simulink model "Aircraft_Simulator_final_"  (R2019b)
settings: Solver=ode4  StartTime=0.0  StopTime=tfinal  FixedStep=dt  RelTol=1e-3
values from neighbouring files (symbols this model uses):
  A_2D = [Yv, -(1-Yr/u0) ... (first row only)    [Approximations.m]
  A_DR = [Yv, 0, -1 ... (first row only)    [Approximations.m]
  A_FL = [Xu, Xw, -w0, -g*cos(theta0) ... (first row only)    [Approximations.m]
  A_lat = [Yb/Vto, (Yp+w0)/Vto, (Yr-u0)/Vto, (g*cos(theta0))/Vto, 0 ... (first row only)    [Approximations.m]
  A_LP = [Xu+w0*Zu/(Zq+u0),          -g*cos(theta0)-w0*g*sin(theta0)/(Zq+u0) ... (first row only)    [Approximations.m]
  A_RO = [Lp_dash]    [Approximations.m]
  A_SP = [Zw/(1-Zwdot), (Zq+u0)/(1-Zwdot) ... (first row only)    [Approximations.m]
  A_Sp = [Lp_dash, Lr_dash, 0 ... (first row only)    [Approximations.m]
  B_2D = [Yda_star, Ydr_star ... (first row only)    [Approximations.m]
  B_DR = [Yda_star, Ydr_star ... (first row only)    [Approximations.m]
  B_FL = [Xde, Xdth ... (first row only)    [Approximations.m]
  B_lat = [Yda_star, Ydr_star ... (first row only)    [Approximations.m]
  B_LP = [Xde+w0*Zde/(Zq+u0), Xdth+w0*Zdth/(Zq+u0) ... (first row only)    [Approximations.m]
  B_RO = [Lda_dash]    [Approximations.m]
  B_SP = [Zde/(1-Zwdot), Zdth/(1-Zwdot) ... (first row only)    [Approximations.m]
  B_Sp = [Lda_dash  Ldr_dash ... (first row only)    [Approximations.m]
  C_2D = eye(2)    [Approximations.m]
  C_DR = eye(3)    [Approximations.m]
  C_FL = eye(4)    [Approximations.m]
  C_lat = eye(5)    [Approximations.m]
  C_LP = eye(2)    [Approximations.m]
  C_RO = eye(1)    [Approximations.m]
  C_SP = eye(2)    [Approximations.m]
  C_Sp = eye(3)    [Approximations.m]
  D_2D = zeros(2)    [Approximations.m]
  D_DR = zeros(3,2)    [Approximations.m]
  D_FL = zeros(4,2)    [Approximations.m]
  D_lat = zeros(5,2)    [Approximations.m]
  D_LP = zeros(2)    [Approximations.m]
  D_RO = zeros(1)    [Approximations.m]
  D_SP = zeros(2,2)    [Approximations.m]
  D_Sp = zeros(3,2)    [Approximations.m]
  da = da(k)*pi/180    [Task4MainCode.m]
  de = 0    [Task4MainCode.m]
  dr = dr(k)*pi/180    [Task4MainCode.m]    (also in afModel.m = cuStates(6)-states0(6))
  dth = 0    [Task4MainCode.m]
undefined symbols (not defined in the file or in its folder): aircraft_data, s0
settings Model: Creator=yossef  LastModifiedBy=Yousef
settings DataIOCC: ReturnWorkspaceOutputs=off
settings DebuggingCC: ArithmeticOperatorsInVariantConditions=warning
settings SFSimCC: SimUseLocalCustomCode=off  CustomCodeUndefinedFunction=UseInterfaceOnly
settings RTWCC: RTWUseLocalCustomCode=off

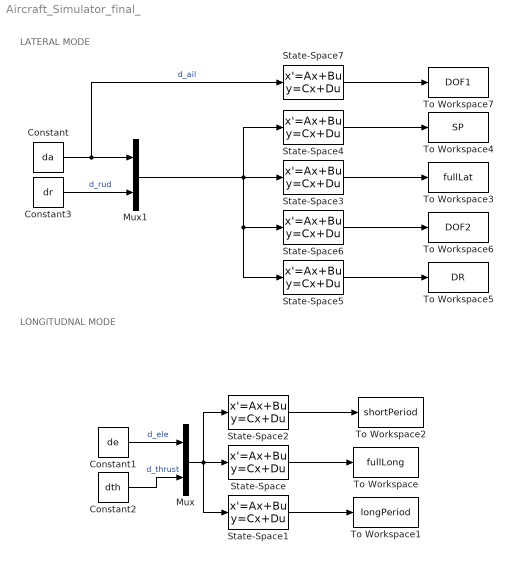
== system Aircraft_Simulator_final_ ==
  note: LONGITUDNAL MODE
  note: LATERAL MODE
  Constant : Constant  Value=da
  Constant1 : Constant  Value=de
  Constant2 : Constant  Value=dth
  Constant3 : Constant  Value=dr
  Mux : Mux  Inputs=2
  Mux1 : Mux  Inputs=2
  State-Space : StateSpace  A=A_FL  B=B_FL  C=C_FL  D=D_FL  InitialCondition=[s0(1),s0(3),s0(5),s0(8)]
  State-Space1 : StateSpace  A=A_LP  B=B_LP  C=C_LP  D=D_LP  InitialCondition=[s0(1),s0(8)]
  State-Space2 : StateSpace  A=A_SP  B=B_SP  C=C_SP  D=D_SP  InitialCondition=[s0(3),s0(5)]
  State-Space3 : StateSpace  A=A_lat  B=B_lat  C=C_lat  D=D_lat  InitialCondition=[aircraft_data(20),s0(4),s0(6),s0(7),s0(9)]
  State-Space4 : StateSpace  A=A_Sp  B=B_Sp  C=C_Sp  D=D_Sp  InitialCondition=[s0(4),s0(6),s0(7)]
  State-Space5 : StateSpace  A=A_DR  B=B_DR  C=C_DR  D=D_DR  InitialCondition=[aircraft_data(20),s0(4),s0(6)]
  State-Space6 : StateSpace  A=A_2D  B=B_2D  C=C_2D  D=D_2D  InitialCondition=[aircraft_data(20),s0(6)]
  State-Space7 : StateSpace  A=A_RO  B=B_RO  C=C_RO  D=D_RO  InitialCondition=[s0(4)]
  To Workspace : ToWorkspace  VariableName=fullLong  SampleTime=-1
      settings: Save2DSignal=2-D array (concatenate along first dimension)
  To Workspace1 : ToWorkspace  VariableName=longPeriod  SampleTime=-1
      settings: Save2DSignal=2-D array (concatenate along first dimension)
  To Workspace2 : ToWorkspace  VariableName=shortPeriod  SampleTime=-1
      settings: Save2DSignal=2-D array (concatenate along first dimension)
  To Workspace3 : ToWorkspace  VariableName=fullLat  SampleTime=-1
      settings: Save2DSignal=2-D array (concatenate along first dimension)
  To Workspace4 : ToWorkspace  VariableName=SP  SampleTime=-1
      settings: Save2DSignal=2-D array (concatenate along first dimension)
  To Workspace5 : ToWorkspace  VariableName=DR  SampleTime=-1
      settings: Save2DSignal=2-D array (concatenate along first dimension)
  To Workspace6 : ToWorkspace  VariableName=DOF2  SampleTime=-1
      settings: Save2DSignal=2-D array (concatenate along first dimension)
  To Workspace7 : ToWorkspace  VariableName=DOF1  SampleTime=-1
      settings: Save2DSignal=2-D array (concatenate along first dimension)
  wires:
  State-Space7/1 -> To Workspace7/1
  State-Space6/1 -> To Workspace6/1
  Constant3/1 -> Mux1/2  "d_rud"
  Mux1/1 -> State-Space6/1, State-Space5/1, State-Space3/1, State-Space4/1
  Constant/1 -> State-Space7/1, Mux1/1  "d_ail"
  State-Space4/1 -> To Workspace4/1
  State-Space5/1 -> To Workspace5/1
  State-Space3/1 -> To Workspace3/1
  Constant2/1 -> Mux/2  "d_thrust"
  State-Space2/1 -> To Workspace2/1
  State-Space/1 -> To Workspace/1
  Constant1/1 -> Mux/1  "d_ele"
  Mux/1 -> State-Space2/1, State-Space/1, State-Space1/1
  State-Space1/1 -> To Workspace1/1
